simulink model "FuelCellElectricSystem"  (R2026b)
settings: Solver=VariableStepAuto
settings Model: ModifiedByFormat=The MathWorks, Inc.  Creator=The MathWorks, Inc.  LastModifiedBy=The MathWorks, Inc.
settings SolverCC: DateTimeAtSimulationTimeZero=[]
settings OptimizationCC: ReuseModelBlockBuffer=off
settings RTWCC: DLArmComputeVersion=19.05
settings SimscapeCC: SimscapeUseEnergyAccounting=off

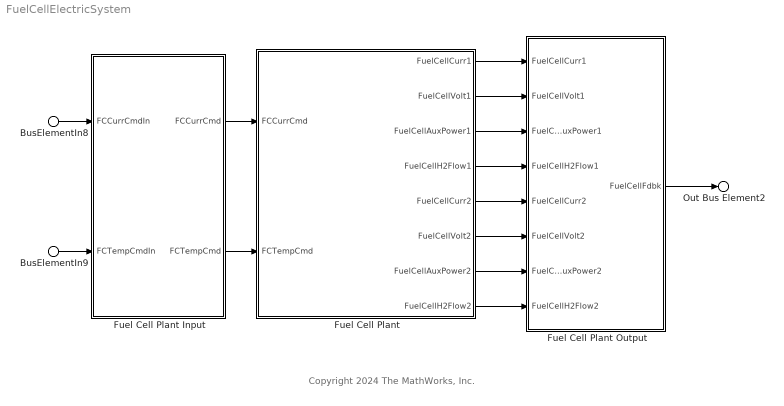
== system FuelCellElectricSystem ==
  note: Copyright 2024 The MathWorks, Inc.
  BusElementIn8 : Inport  PortName=Cntrl  Element=Vcu.FuelCellCurrCmd
  BusElementIn9 : Inport  PortName=Cntrl  Element=Vcu.FuelCellCurrCmd
  Fuel Cell Plant : Subsystem
  Fuel Cell Plant Input : Subsystem
      settings: CopyFcn=set_param(gcb,'BackgroundColor','white');
  Fuel Cell Plant Output : Subsystem
  Out Bus Element2 : Outport  PortName=FuelCell
  wires:
  BusElementIn8/1 -> Fuel Cell Plant Input/1(FCCurrCmdIn)
  BusElementIn9/1 -> Fuel Cell Plant Input/2(FCTempCmdIn)
  Fuel Cell Plant Output/1(FuelCellFdbk) -> Out Bus Element2/1
  Fuel Cell Plant Input/2(FCTempCmd) -> Fuel Cell Plant/2(FCTempCmd)
  Fuel Cell Plant Input/1(FCCurrCmd) -> Fuel Cell Plant/1(FCCurrCmd)
  Fuel Cell Plant/1(FuelCellCurr1) -> Fuel Cell Plant Output/1(FuelCellCurr1)
  Fuel Cell Plant/2(FuelCellVolt1) -> Fuel Cell Plant Output/2(FuelCellVolt1)
  Fuel Cell Plant/3(FuelCellAuxPower1) -> Fuel Cell Plant Output/3(FuelCellAuxPower1)
  Fuel Cell Plant/4(FuelCellH2Flow1) -> Fuel Cell Plant Output/4(FuelCellH2Flow1)
  Fuel Cell Plant/5(FuelCellCurr2) -> Fuel Cell Plant Output/5(FuelCellCurr2)
  Fuel Cell Plant/6(FuelCellVolt2) -> Fuel Cell Plant Output/6(FuelCellVolt2)
  Fuel Cell Plant/7(FuelCellAuxPower2) -> Fuel Cell Plant Output/7(FuelCellAuxPower2)
  Fuel Cell Plant/8(FuelCellH2Flow2) -> Fuel Cell Plant Output/8(FuelCellH2Flow2)

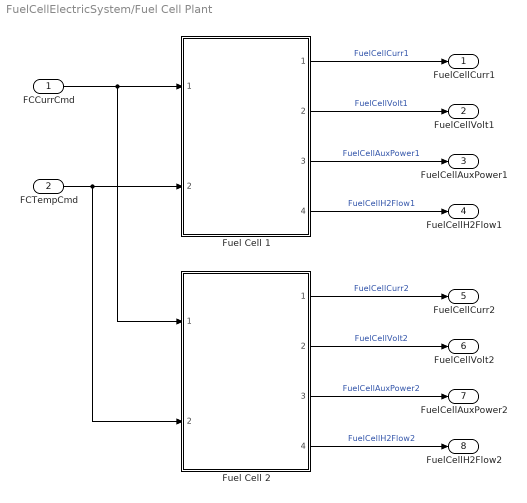
== system FuelCellElectricSystem/Fuel Cell Plant ==
  FCCurrCmd : Inport
  FCTempCmd : Inport  Port=2
  Fuel Cell 1 : Subsystem  ReferencedSubsystem=FuelCellCore
  Fuel Cell 2 : Subsystem  ReferencedSubsystem=FuelCellCore
  FuelCellCurr1 : Outport
  FuelCellVolt1 : Outport  Port=2
  FuelCellAuxPower1 : Outport  Port=3
  FuelCellH2Flow1 : Outport  Port=4
  FuelCellCurr2 : Outport  Port=5
  FuelCellVolt2 : Outport  Port=6
  FuelCellAuxPower2 : Outport  Port=7
  FuelCellH2Flow2 : Outport  Port=8
  wires:
  Fuel Cell 1/4 -> FuelCellH2Flow1/1  "FuelCellH2Flow1"
  FCTempCmd/1 -> Fuel Cell 2/2, Fuel Cell 1/2
  Fuel Cell 1/1 -> FuelCellCurr1/1  "FuelCellCurr1"
  FCCurrCmd/1 -> Fuel Cell 2/1, Fuel Cell 1/1
  Fuel Cell 2/2 -> FuelCellVolt2/1  "FuelCellVolt2"
  Fuel Cell 2/1 -> FuelCellCurr2/1  "FuelCellCurr2"
  Fuel Cell 1/3 -> FuelCellAuxPower1/1  "FuelCellAuxPower1"
  Fuel Cell 2/3 -> FuelCellAuxPower2/1  "FuelCellAuxPower2"
  Fuel Cell 2/4 -> FuelCellH2Flow2/1  "FuelCellH2Flow2"
  Fuel Cell 1/2 -> FuelCellVolt1/1  "FuelCellVolt1"

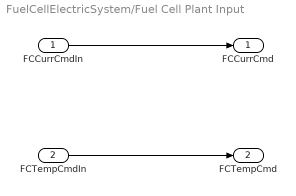
== system FuelCellElectricSystem/Fuel Cell Plant Input ==
  FCCurrCmdIn : Inport
  FCTempCmdIn : Inport  Port=2
  FCCurrCmd : Outport  VectorParamsAs1DForOutWhenUnconnected=off
  FCTempCmd : Outport  Port=2  VectorParamsAs1DForOutWhenUnconnected=off
  wires:
  FCTempCmdIn/1 -> FCTempCmd/1
  FCCurrCmdIn/1 -> FCCurrCmd/1

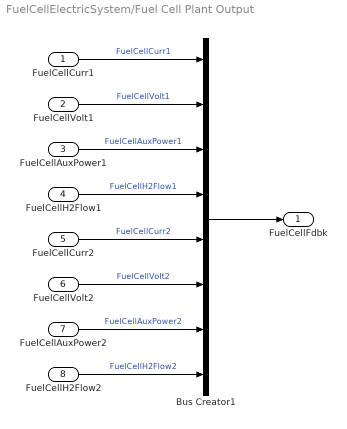
== system FuelCellElectricSystem/Fuel Cell Plant Output ==
  FuelCellCurr1 : Inport
  FuelCellVolt1 : Inport  Port=2
  FuelCellAuxPower1 : Inport  Port=3
  FuelCellH2Flow1 : Inport  Port=4
  FuelCellCurr2 : Inport  Port=5
  FuelCellVolt2 : Inport  Port=6
  FuelCellAuxPower2 : Inport  Port=7
  FuelCellH2Flow2 : Inport  Port=8
  Bus Creator1 : BusCreator  Inputs=8
  FuelCellFdbk : Outport
  wires:
  Bus Creator1/1 -> FuelCellFdbk/1
  FuelCellCurr1/1 -> Bus Creator1/1  "FuelCellCurr1"
  FuelCellVolt1/1 -> Bus Creator1/2  "FuelCellVolt1"
  FuelCellAuxPower1/1 -> Bus Creator1/3  "FuelCellAuxPower1"
  FuelCellH2Flow1/1 -> Bus Creator1/4  "FuelCellH2Flow1"
  FuelCellCurr2/1 -> Bus Creator1/5  "FuelCellCurr2"
  FuelCellVolt2/1 -> Bus Creator1/6  "FuelCellVolt2"
  FuelCellAuxPower2/1 -> Bus Creator1/7  "FuelCellAuxPower2"
  FuelCellH2Flow2/1 -> Bus Creator1/8  "FuelCellH2Flow2"
